simulink model "untitled1"  (R2024a)
settings: Solver=VariableStepAuto  StartTime=0.0  StopTime=0.25  RelTol=1e-3
values from neighbouring files (symbols this model uses):
  den = [1 2 3]    [Jara_Ivan_T2.m]    (also in dos.m = [1, R/L, 1/(L*Cap)]; uno.m = [1 2*xi*wn wn^2]; untitled.m = [1 R/L 1/(L*Cap)])
  Kd = 0.01    [dos.m]    (also in untitled.m)
  Ki = 1000    [dos.m]    (also in tres.m = 9.43; untitled.m)
  Kp = 10    [dos.m]    (also in untitled.m)
  num = [3]    [Jara_Ivan_T2.m]    (also in dos.m = 45454.5454545; uno.m = 1; untitled.m = 45454.5454545)
settings Model: Creator=ivanc  LastModifiedBy=ivanc

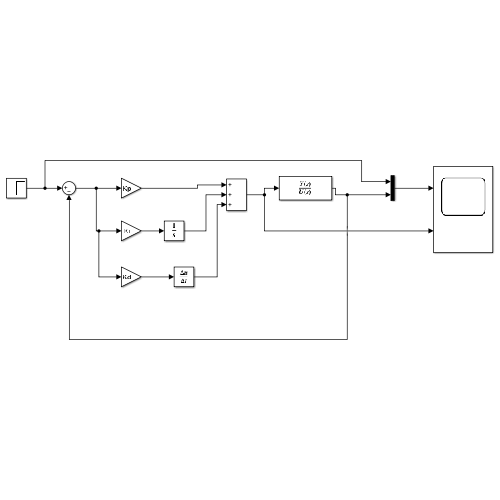
[thumbnail: Simulink's stored preview of the top-level diagram]
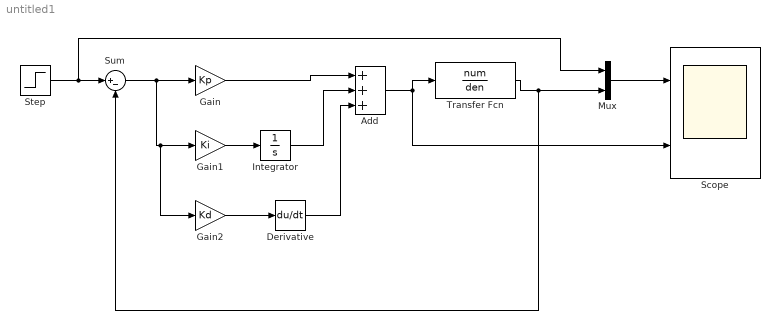
== system untitled1 ==
  Add : Sum  Inputs=+++
  Derivative : Derivative
  Gain : Gain  Gain=Kp
  Gain1 : Gain  Gain=Ki
  Gain2 : Gain  Gain=Kd
  Integrator : Integrator
  Mux : Mux  Inputs=2
  Scope : Scope  NumInputPorts=2
  Step : Step  Time=0.01  After=5  SampleTime=0
  Sum : Sum  Inputs=|+-
  Transfer Fcn : TransferFcn  Numerator=num  Denominator=den
  wires:
  Transfer Fcn/1 -> Mux/2, Sum/2
  Step/1 -> Mux/1, Sum/1
  Sum/1 -> Gain2/1, Gain1/1, Gain/1
  Gain1/1 -> Integrator/1
  Add/1 -> Transfer Fcn/1, Scope/2
  Gain/1 -> Add/1
  Integrator/1 -> Add/2
  Mux/1 -> Scope/1
  Gain2/1 -> Derivative/1
  Derivative/1 -> Add/3
